simulink model "freq_divider_10"  (R2019a)
settings: Solver=VariableStepAuto  StartTime=0.0  StopTime=30  MaxStep=0.1  RelTol=1e-3
libraries: simulink_extras x6
settings Model: Creator=何泽楷  LastModifiedBy=何泽楷
settings OptimizationCC: BooleanDataType=off

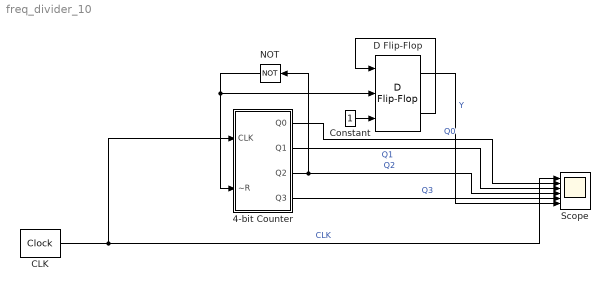
== system freq_divider_10 ==
  4-bit Counter : Subsystem
  CLK : simulink_extras/Flip Flops/Clock  period=1
  Constant : Constant
  D Flip-Flop : simulink_extras/Flip Flops/D Flip-Flop
      settings: SourceProductName=Simulink
  NOT : Logic  Operator=NOT  IconShape=distinctive  AllPortsSameDT=off
  Scope : Scope  NumInputPorts=6
  wires:
  CLK/1 -> Scope/1, 4-bit Counter/1(CLK)  "CLK"
  4-bit Counter/1(Q0) -> Scope/2  "Q0"
  4-bit Counter/2(Q1) -> Scope/3  "Q1"
  4-bit Counter/3(Q2) -> NOT/1, Scope/4  "Q2"
  4-bit Counter/4(Q3) -> Scope/5  "Q3"
  Constant/1 -> D Flip-Flop/3
  NOT/1 -> 4-bit Counter/2(~R), D Flip-Flop/2
  D Flip-Flop/2 -> D Flip-Flop/1
  D Flip-Flop/1 -> Scope/6  "Y"

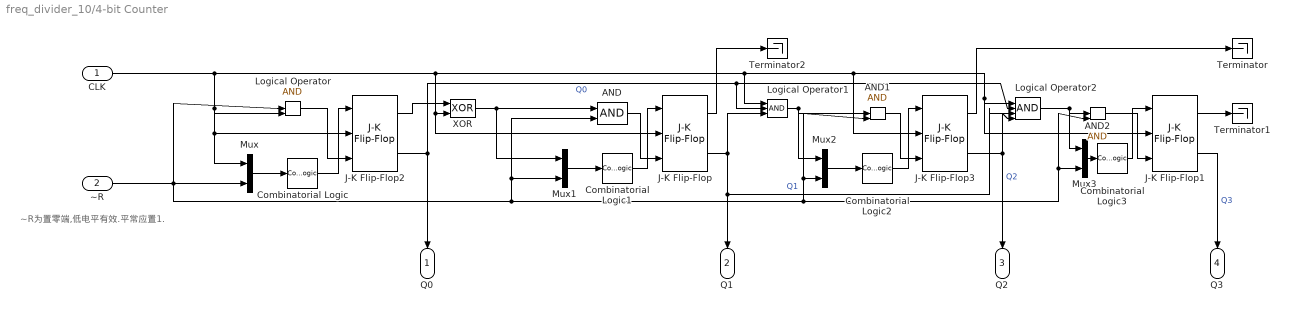
== system freq_divider_10/4-bit Counter ==
  note: ~R为置零端,低电平有效.平常应置1.
  CLK : Inport
  ~R : Inport  Port=2  OutDataTypeStr=double
  AND : Logic  IconShape=distinctive  AllPortsSameDT=off
  AND1 : Logic  IconShape=distinctive  AllPortsSameDT=off
  AND2 : Logic  IconShape=distinctive  AllPortsSameDT=off
  Combinatorial Logic{,1..3} (4 alike) : CombinatorialLogic  TruthTable=[1;0;1;1];
  J-K Flip-Flop{,1..3} (4 alike) : simulink_extras/Flip Flops/J-K Flip-Flop  initial_condition=0
      settings: SourceProductName=Simulink
  Logical Operator : Logic  IconShape=distinctive  AllPortsSameDT=off
  Logical Operator1 : Logic  Inputs=3  IconShape=distinctive  AllPortsSameDT=off
  Logical Operator2 : Logic  Inputs=4  IconShape=distinctive  AllPortsSameDT=off
  Mux{,1..3} (4 alike) : Mux  Inputs=2
  Terminator : Terminator
  Terminator1 : Terminator
  Terminator2 : Terminator
  XOR : Logic  Operator=XOR  IconShape=distinctive  AllPortsSameDT=off
  Q0 : Outport
  Q1 : Outport  Port=2
  Q2 : Outport  Port=3
  Q3 : Outport  Port=4
  wires:
  J-K Flip-Flop2/2 -> Q0/1, Logical Operator2/2, Logical Operator1/2  "Q0"
  Logical Operator1/1 -> AND1/1, Mux2/1
  J-K Flip-Flop2/1 -> XOR/1
  J-K Flip-Flop3/2 -> Q2/1, Logical Operator2/4  "Q2"
  J-K Flip-Flop/2 -> Q1/1, Logical Operator2/3, Logical Operator1/3  "Q1"
  J-K Flip-Flop1/2 -> Q3/1  "Q3"
  Logical Operator/1 -> J-K Flip-Flop2/3
  CLK/1 -> Mux/1, J-K Flip-Flop2/2, Logical Operator/2, J-K Flip-Flop/2, XOR/2, J-K Flip-Flop1/2, Logical Operator2/1, J-K Flip-Flop3/2, Logical Operator1/1
  Combinatorial Logic/1 -> J-K Flip-Flop2/1
  Mux/1 -> Combinatorial Logic/1
  XOR/1 -> Mux1/1, AND/1
  Mux1/1 -> Combinatorial Logic1/1
  Combinatorial Logic1/1 -> J-K Flip-Flop/1
  Mux2/1 -> Combinatorial Logic2/1
  Combinatorial Logic2/1 -> J-K Flip-Flop3/1
  ~R/1 -> AND/2, Mux1/2, AND1/2, Mux2/2, Mux3/2, AND2/2, Logical Operator/1, Mux/2
  Logical Operator2/1 -> Mux3/1, AND2/1
  Mux3/1 -> Combinatorial Logic3/1
  Combinatorial Logic3/1 -> J-K Flip-Flop1/1
  AND/1 -> J-K Flip-Flop/3
  AND1/1 -> J-K Flip-Flop3/3
  AND2/1 -> J-K Flip-Flop1/3
  J-K Flip-Flop3/1 -> Terminator/1
  J-K Flip-Flop1/1 -> Terminator1/1
  J-K Flip-Flop/1 -> Terminator2/1
